simulink model "level_flight"  (R2015b)
settings: Solver=VariableStepAuto  StartTime=0.0  StopTime=300  RelTol=1e-3
settings Model: Creator=Pramod  LastModifiedBy=Pramod

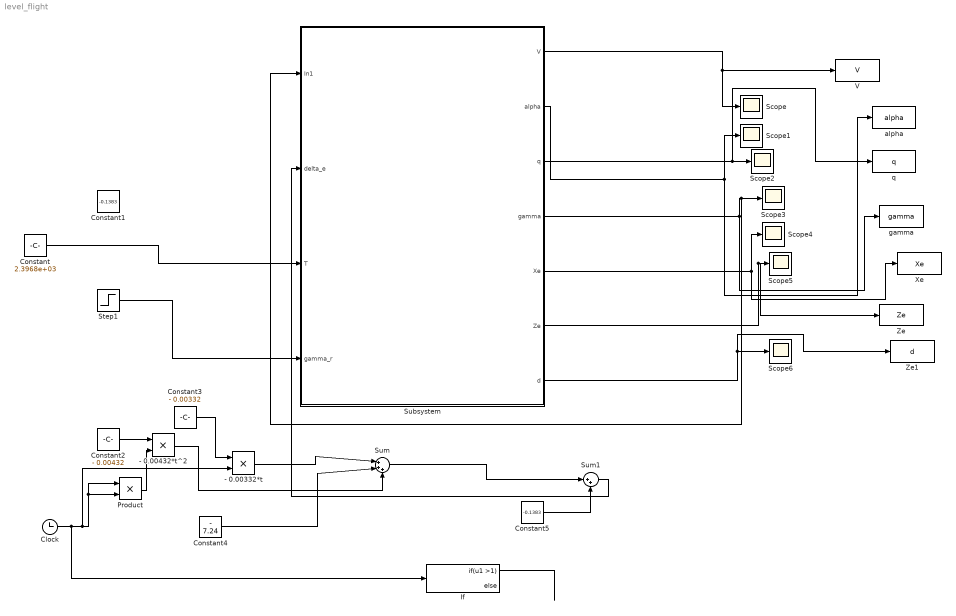
== system level_flight ==
  - 0.00332*t : Product
  - 0.00432*t^2 : Product
  Clock : Clock
  Constant : Constant  Value=2.3968e+03
  Constant1 : Constant  Value=-0.1383
  Constant2 : Constant  Value=- 0.00432
  Constant3 : Constant  Value=- 0.00332
  Constant4 : Constant  Value=- 7.24
  Constant5 : Constant  Value=-0.1383
  If : If  IfExpression=u1 >1
  Product : Product
  Scope{,1..6} (7 alike) : Scope
  Step1 : Step  Time=5  After=-2.5*pi/180  SampleTime=0
  Subsystem : Subsystem
  Sum : Sum  Inputs=|+++
  Sum1 : Sum  Inputs=|++
  V : ToWorkspace  VariableName=V  SaveFormat=Timeseries  SampleTime=-1
  Xe : ToWorkspace  VariableName=Xe  SaveFormat=Timeseries  SampleTime=-1
  Ze : ToWorkspace  VariableName=Ze  SaveFormat=Timeseries  SampleTime=-1
  Ze1 : ToWorkspace  VariableName=d  SaveFormat=Timeseries  SampleTime=-1
  alpha : ToWorkspace  VariableName=alpha  SaveFormat=Timeseries  SampleTime=-1
  gamma : ToWorkspace  VariableName=gamma  SaveFormat=Timeseries  SampleTime=-1
  q : ToWorkspace  VariableName=q  SaveFormat=Timeseries  SampleTime=-1
  wires:
  Subsystem/2(alpha) -> alpha/1, Scope1/1
  Subsystem/3(q) -> q/1, Scope2/1
  Subsystem/5(Xe) -> Scope4/1, Xe/1
  Subsystem/7(d) -> Ze1/1, Scope6/1
  Subsystem/4(gamma) -> Subsystem/1(In1), Scope3/1, gamma/1
  Subsystem/6(Ze) -> Ze/1, Scope5/1
  Subsystem/1(V) -> Scope/1, V/1
  Step1/1 -> Subsystem/4(gamma_r)
  Constant/1 -> Subsystem/3(T)
  Clock/1 -> If/1, - 0.00332*t/2, Product/2, Product/1
  Constant2/1 -> - 0.00432*t^2/1
  Product/1 -> - 0.00432*t^2/2
  Constant3/1 -> - 0.00332*t/1
  - 0.00332*t/1 -> Sum/1
  Constant4/1 -> Sum/2
  - 0.00432*t^2/1 -> Sum/3
  Sum/1 -> Sum1/1
  Constant5/1 -> Sum1/2
  Sum1/1 -> Subsystem/2(delta_e)
  If/1 -> ?

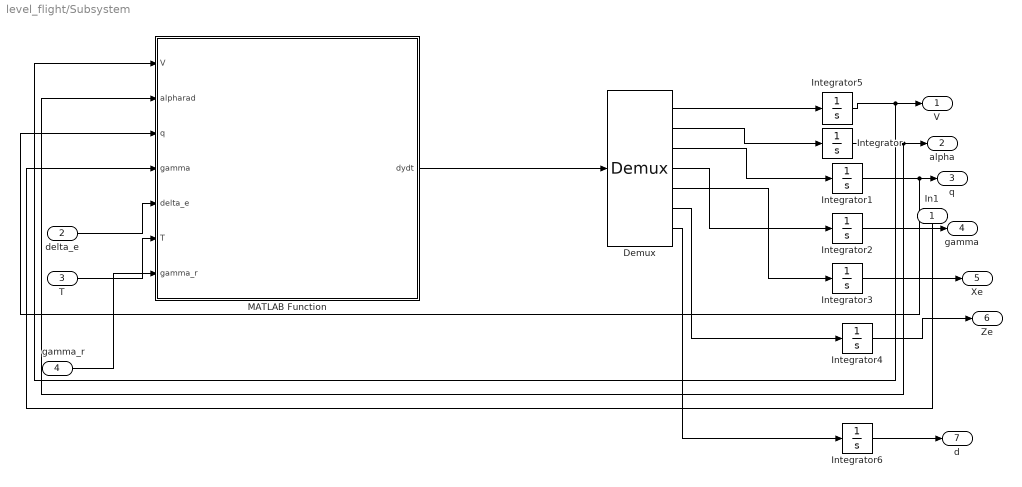
== system level_flight/Subsystem ==
  In1 : Inport
  delta_e : Inport  Port=2
  T : Inport  Port=3
  gamma_r : Inport  Port=4
  Demux : Demux  Outputs=7
  Integrator : Integrator  InitialCondition=4.8*pi/180
  Integrator1 : Integrator  InitialCondition=0.01
  Integrator2 : Integrator
  Integrator3 : Integrator  InitialCondition=1500
  Integrator4 : Integrator
  Integrator5 : Integrator  InitialCondition=42
  Integrator6 : Integrator
  MATLAB Function : MATLAB Function  TreatAsAtomicUnit=on
  V : Outport
  alpha : Outport  Port=2
  q : Outport  Port=3
  gamma : Outport  Port=4
  Xe : Outport  Port=5
  Ze : Outport  Port=6
  d : Outport  Port=7
  wires:
  delta_e/1 -> MATLAB Function/5(delta_e)
  MATLAB Function/1(dydt) -> Demux/1
  T/1 -> MATLAB Function/6(T)
  Integrator3/1 -> Xe/1
  Integrator2/1 -> gamma/1
  Integrator4/1 -> Ze/1
  Demux/2 -> Integrator/1
  Demux/4 -> Integrator2/1
  Demux/3 -> Integrator1/1
  Integrator5/1 -> V/1, MATLAB Function/1(V)
  Demux/6 -> Integrator4/1
  Demux/1 -> Integrator5/1
  Integrator1/1 -> q/1, MATLAB Function/3(q)
  Demux/5 -> Integrator3/1
  Integrator/1 -> alpha/1, MATLAB Function/2(alpharad)
  gamma_r/1 -> MATLAB Function/7(gamma_r)
  Demux/7 -> Integrator6/1
  In1/1 -> MATLAB Function/4(gamma)
  Integrator6/1 -> d/1

== matlab function level_flight/Subsystem/MATLAB Function ==
  data: V input; dydt output; alpharad input; q input; gamma input; delta_e input; T input; gamma_r input
function dydt = fcn(V,alpharad,q,gamma,delta_e,T,gamma_r)
g = 9.8;
rho = 1.225;
%q=0
%gamma=0 % for level flight
m = 1043.26;
C_bar = 1.493;
b = 10.911;
S_ref = 16.1651;
%delta_e= -0.1383;
%T=    2.3968e+03
% if t==0 && t<=100
% delta_e= -0.1383;
% end
%  if t>=101&&t<=102
%        delta_e= -0.1383-(pi/180);
%     end
%     if t>103 && t<=200
%      delta_e= -0.1383;
%     end
%     
%     

  %T=  2.3968e+03
%T=1.5206e+03

%T=1.2109e+04
%T= 2.4989e+03;
% if t==0 && t<=100
% T=  -2.4989e+03;
% end
%  if t>=101&&t<=111
%         T=  -2.4989e+03*1.1;
%     end
%     if t>103 && t<=200
%        T=-2.4989e+03;
%     end
%  if t>=101&&t<=105
%         T=  1.2109e+04+1*10^4;
%     end
%     if t>103 && t<=200
%         T=1.2109e+04;
%      end


C_L_0 = 0.25;
C_L_alpha = 4.47;
C_L_q = 1.7;
C_L_delta_e = 0.3476;

% Ignore all other C_D derivatives excluding C_D_0
% Use C_D = C_D_0 + k*C_L^2

C_D_0 = 0.036;
k = 0.3;

C_Y_beta = -0.31;
C_Y_p = -0.037;
C_Y_r = 0.21;
C_Y_delta_a = 0;

C_l_beta = -0.089;
C_l_p = -0.47;
C_l_r = 0.096;
C_l_delta_a = -0.09;
C_l_delta_r = 0.0147;

C_M_0 = -0.02;
C_M_alpha = -1.8;
C_M_alpha_dot = -12.4;
C_M_delta_e = -1.28;

C_N_beta = 0.065;
C_N_p = -0.03;
C_N_r = -0.99;
C_N_delta_a = -0.0053;
C_N_delta_r = -0.0657;
I_yy = 1824.93;
%delta_erad=-( C_M_0 +C_M_alpha*alpharad)/C_M_delta_e
C_L = C_L_0 + C_L_alpha*alpharad +   C_L_delta_e*delta_e
C_D = C_D_0 + k*C_L^2
C_M = C_M_0 + C_M_alpha*alpharad +  C_M_delta_e*delta_e
C_X = -C_D*cos(alpharad) + C_L*sin(alpharad)
C_Z = -C_D*sin(alpharad) - C_L*cos(alpharad)

dydt=zeros(7,1)
dydt(1)=1/(m)*(T*cos(alpharad)-m*g*sin(gamma)-.5*rho*V^2*S_ref*C_D);
dydt(2)=q-(-g/V+.5*rho*V^2*S_ref*C_L/(m*V)+T*sin(alpharad)/(m*V));
dydt(3)=1/(2*I_yy)*rho*(V^2)*S_ref*C_bar*C_M
dydt(4)=q;
dydt(5)=V*cos(gamma);
dydt(6)=-V*sin(gamma);
dydt(7)=60*sin(gamma-gamma_r)
